simulink model "zad3_3_1_e"  (Simulink 6.5)
settings: Solver=ode45  StartTime=0.0  StopTime=10.0  RelTol=1e-3
settings Model: Creator=rr44283  LastModifiedBy=rr44283

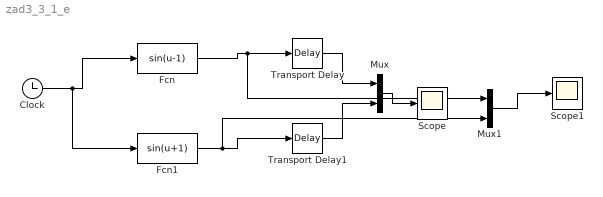
== system zad3_3_1_e ==
  Clock : Clock
      settings: Decimation=10
  Fcn : Fcn  Expr=sin(u-1)
  Fcn1 : Fcn  Expr=sin(u+1)
  Mux : Mux  Inputs=2
  Mux1 : Mux  Inputs=2
  Scope : Scope
  Scope1 : Scope
  Transport Delay : TransportDelay
  Transport Delay1 : TransportDelay
  wires:
  Clock/1 -> Fcn/1, Fcn1/1
  Fcn/1 -> Transport Delay/1, Mux1/1
  Fcn1/1 -> Transport Delay1/1, Mux1/2
  Transport Delay/1 -> Mux/1
  Transport Delay1/1 -> Mux/2
  Mux/1 -> Scope/1
  Mux1/1 -> Scope1/1
